simulink model "plant_comp"  (R2025b)
settings: Solver=VariableStepAuto  StartTime=0.0  StopTime=13  RelTol=1e-3
settings Model: Creator=ardag  LastModifiedBy=ardag

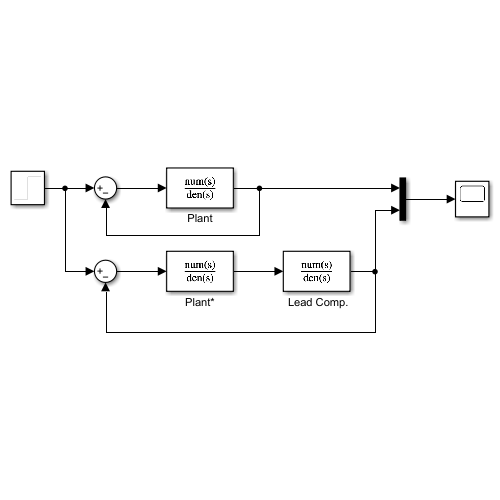
[thumbnail: Simulink's stored preview of the top-level diagram]
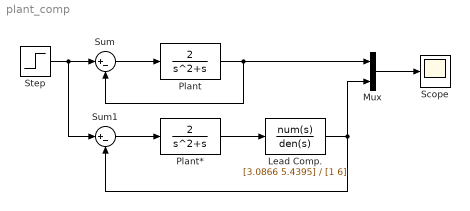
== system plant_comp ==
  " Lead Comp." : TransferFcn  Numerator=[3.0866 5.4395]  Denominator=[1 6]
  Mux : Mux  Inputs=2
  Plant : TransferFcn  Numerator=[2]  Denominator=[1 1 0]
  Plant* : TransferFcn  Numerator=[2]  Denominator=[1 1 0]
  Scope : Scope
      settings: ActiveDisplayYMinimum=-0.16310623970245186  ActiveDisplayYMaximum=1.467956157322067
  Step : Step  Time=0  SampleTime=0
  Sum : Sum  Inputs=|+-
  Sum1 : Sum  Inputs=|+-
  wires:
  Step/1 -> Sum1/1, Sum/1
  Sum/1 -> Plant/1
  Mux/1 -> Scope/1
  Plant/1 -> Sum/2, Mux/1
  Sum1/1 -> Plant*/1
  Plant*/1 -> " Lead Comp."/1
  " Lead Comp."/1 -> Mux/2, Sum1/2
